simulink model "control_tester"  (R2024b)
settings: Solver=FixedStepAuto  StartTime=0.0  StopTime=40  FixedStep=0.01  RelTol=1e-3
settings Model: Creator=Emil  LastModifiedBy=Emil

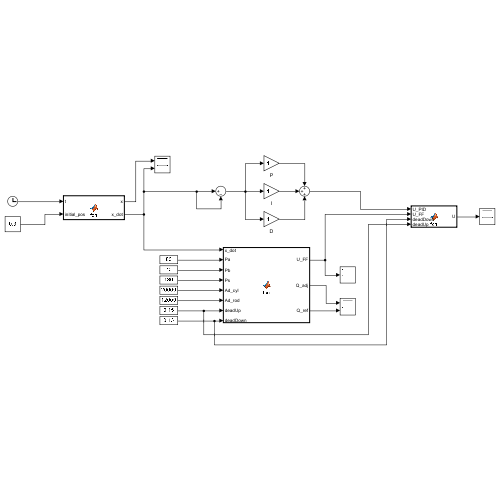
[thumbnail: Simulink's stored preview of the top-level diagram]
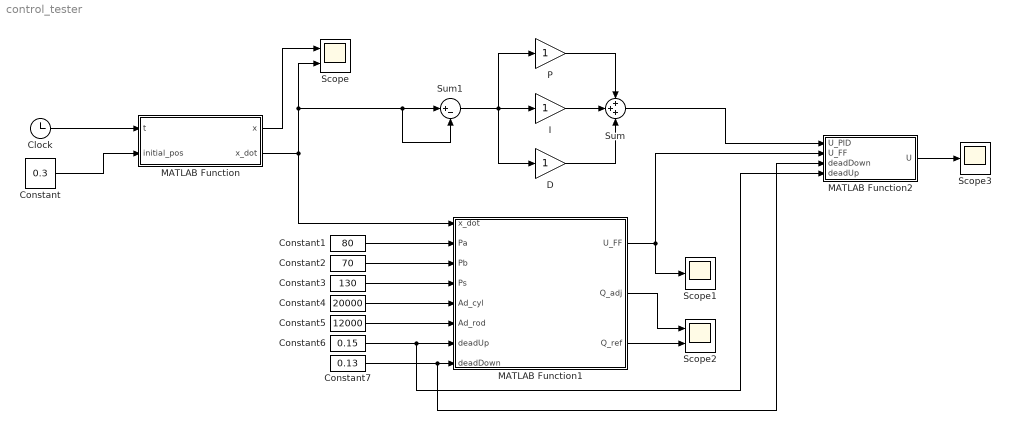
== system control_tester ==
  Clock : Clock
  Constant : Constant  Value=0.3
  Constant1 : Constant  Value=80
  Constant2 : Constant  Value=70
  Constant3 : Constant  Value=130
  Constant4 : Constant  Value=20000
  Constant5 : Constant  Value=12000
  Constant6 : Constant  Value=0.15
  Constant7 : Constant  Value=0.13
  D : Gain
  I : Gain
  MATLAB Function : MATLAB Function  TreatAsAtomicUnit=on
  MATLAB Function1 : MATLAB Function  TreatAsAtomicUnit=on
  MATLAB Function2 : MATLAB Function  TreatAsAtomicUnit=on
  P : Gain
  Scope : Scope  NumInputPorts=2
  Scope1 : Scope
  Scope2 : Scope  NumInputPorts=2
  Scope3 : Scope
  Sum : Sum  Inputs=+++
  Sum1 : Sum  Inputs=|+-
  wires:
  Clock/1 -> MATLAB Function/1(t)
  MATLAB Function/1(x) -> Scope/1
  Constant/1 -> MATLAB Function/2(initial_pos)
  MATLAB Function/2(x_dot) -> Sum1/2, Sum1/1, Scope/2, MATLAB Function1/1(x_dot)
  Constant6/1 -> MATLAB Function2/4(deadUp), MATLAB Function1/7(deadUp)
  Constant7/1 -> MATLAB Function2/3(deadDown), MATLAB Function1/8(deadDown)
  Constant5/1 -> MATLAB Function1/6(Ad_rod)
  Constant4/1 -> MATLAB Function1/5(Ad_cyl)
  Constant3/1 -> MATLAB Function1/4(Ps)
  Constant2/1 -> MATLAB Function1/3(Pb)
  Constant1/1 -> MATLAB Function1/2(Pa)
  MATLAB Function1/1(U_FF) -> MATLAB Function2/2(U_FF), Scope1/1
  MATLAB Function1/2(Q_adj) -> Scope2/1
  MATLAB Function1/3(Q_ref) -> Scope2/2
  Sum/1 -> MATLAB Function2/1(U_PID)
  Sum1/1 -> D/1, I/1, P/1
  MATLAB Function2/1(U) -> Scope3/1
  P/1 -> Sum/1
  I/1 -> Sum/2
  D/1 -> Sum/3

== matlab function control_tester/MATLAB Function1 ==
  data: x_dot input; U_FF output; Pa input; Pb input; Ps input; Ad_cyl input; Ad_rod input; deadUp input; deadDown input; Q_adj output; Q_ref output
function [U_FF,Q_adj,Q_ref] = fcn(x_dot, Pa, Pb, Ps, Ad_cyl,Ad_rod,deadUp,deadDown)

dp_0 = 6e5; %Pa
Q_0 = 30/60000; %m^3/s

if x_dot >= 0
    dp = (Ps-Pa)*1e5;
    if dp <=100
        dp = 100;
    end
    Q_ref = Ad_cyl*1e-6 * x_dot;
    Q_adj = Q_ref * sqrt(dp_0/dp);
    U_FF = Q_adj/Q_0;
    U_FF = U_FF*(1-deadUp);
elseif x_dot < 0
    dp = (Ps-Pb)*1e5;
    if dp <=100
        dp = 100;
    end
    Q_ref = Ad_rod*1e-6 * x_dot;
    Q_adj = Q_ref * sqrt(dp_0/dp);
    U_FF = Q_adj/Q_0;
    U_FF = U_FF*(1-deadDown);
else
    U_FF = 0;
    Q_ref = 0;
    Q_adj = 0;
end

Q_ref = Q_ref*60000;
Q_adj = Q_adj*60000;

== matlab function control_tester/MATLAB Function ==
  data: t input; x output; initial_pos input; x_dot output
function [x, x_dot] = fcn(t,initial_pos)

amplitude = 0.1;
median = initial_pos+amplitude;
frekvens = 0.05;

x = median - amplitude * cos(2*pi*frekvens*t);
x_dot = amplitude*2*pi*frekvens*sin(2*pi*frekvens*t);

== matlab function control_tester/MATLAB Function2 ==
  data: U_PID input; U_FF input; U output; deadDown input; deadUp input
function U = fcn(U_PID,U_FF, deadDown, deadUp)
U_adj = U_FF+U_PID;
if U_PID >= 0
    U = U_adj+deadUp;
elseif U_PID < 0
    U = U_adj-deadDown;
else
    U=0;
end
